simulink model "LADRC_Bloque_py"  (R2021a)
settings: Solver=ode8  StartTime=0.0  StopTime=Tsim  FixedStep=0.01  RelTol=1e-3
undefined symbols (not defined in the file or in its folder): Alpha, Kconva, Kconvp, Krad, mcecool, mcehot, mcerad, Rp, Tamb, Vfan
settings Model: Creator=djah0  LastModifiedBy=djah0
settings DataIOCC: ReturnWorkspaceOutputs=off

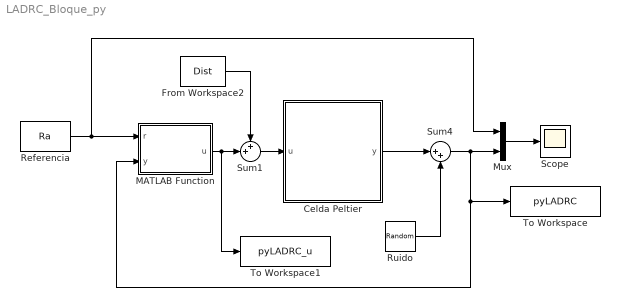
== system LADRC_Bloque_py ==
  Celda Peltier : Subsystem
  From Workspace2 : FromWorkspace  VariableName=Dist
  MATLAB Function : MATLAB Function  TreatAsAtomicUnit=on
  Mux : Mux  Inputs=2
  Referencia : FromWorkspace  VariableName=Ra
  Ruido : RandomNumber  Variance=0.002  Seed=1  SampleTime=0.2
  Scope : Scope
  Sum1 : Sum  Inputs=++|
  Sum4 : Sum  Inputs=|++
  To Workspace : ToWorkspace  VariableName=pyLADRC  SaveFormat=Timeseries  SampleTime=-1
  To Workspace1 : ToWorkspace  VariableName=pyLADRC_u  SaveFormat=Timeseries  SampleTime=-1
  wires:
  Sum1/1 -> Celda Peltier/1(u)
  MATLAB Function/1(u) -> To Workspace1/1, Sum1/2
  From Workspace2/1 -> Sum1/1
  Referencia/1 -> Mux/1, MATLAB Function/1(r)
  Mux/1 -> Scope/1
  Celda Peltier/1(y) -> Sum4/1
  Sum4/1 -> MATLAB Function/2(y), To Workspace/1, Mux/2
  Ruido/1 -> Sum4/2

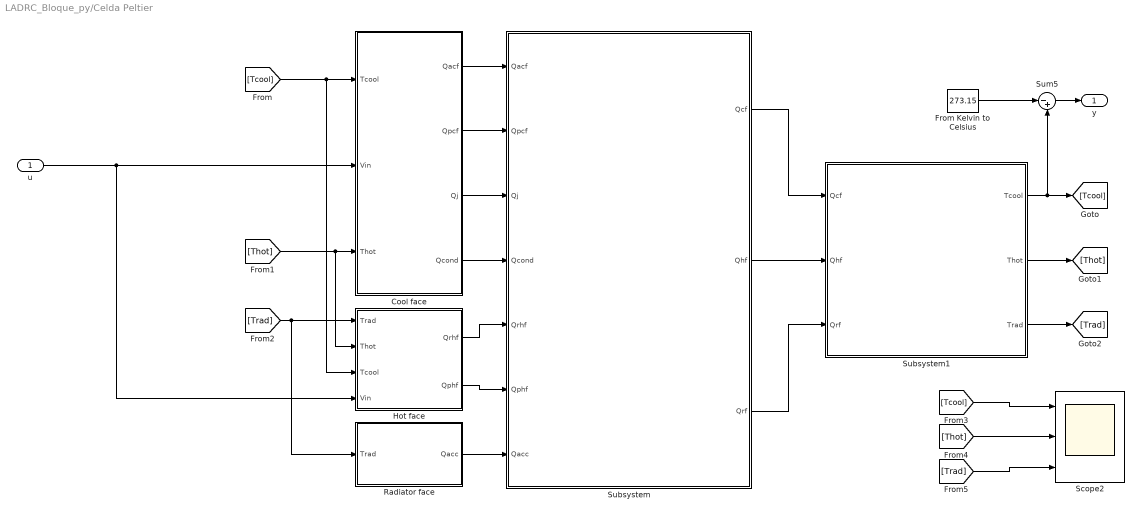
== system LADRC_Bloque_py/Celda Peltier ==
  u : Inport
  Cool face : Subsystem
  From Kelvin to Celsius : Constant  Value=273.15
  Hot face : Subsystem
  Radiator face : Subsystem
  Scope2 : Scope  NumInputPorts=3
  Subsystem : Subsystem
  Subsystem1 : Subsystem
  Sum5 : Sum  Inputs=|-+
  y : Outport  VectorParamsAs1DForOutWhenUnconnected=off
  wires:
  u/1 -> Hot face/4(Vin), Cool face/2(Vin)
  [Tcool] -> Hot face/3(Tcool), Cool face/1(Tcool)
  Subsystem1/1(Tcool) -> [Tcool], Sum5/2
  Radiator face/1(Qacc) -> Subsystem/7(Qacc)
  Subsystem1/3(Trad) -> [Trad]
  [Thot] -> Hot face/2(Thot), Cool face/3(Thot)
  [Trad] -> Hot face/1(Trad), Radiator face/1(Trad)
  Subsystem1/2(Thot) -> [Thot]
  Cool face/2(Qpcf) -> Subsystem/2(Qpcf)
  Cool face/1(Qacf) -> Subsystem/1(Qacf)
  Cool face/3(Qj) -> Subsystem/3(Qj)
  Cool face/4(Qcond) -> Subsystem/4(Qcond)
  Subsystem/1(Qcf) -> Subsystem1/1(Qcf)
  Subsystem/2(Qhf) -> Subsystem1/2(Qhf)
  Subsystem/3(Qrf) -> Subsystem1/3(Qrf)
  Hot face/1(Qrhf) -> Subsystem/5(Qrhf)
  Hot face/2(Qphf) -> Subsystem/6(Qphf)
  Sum5/1 -> y/1
  From Kelvin to Celsius/1 -> Sum5/1
  [Tcool] -> Scope2/1
  [Thot] -> Scope2/2
  [Trad] -> Scope2/3

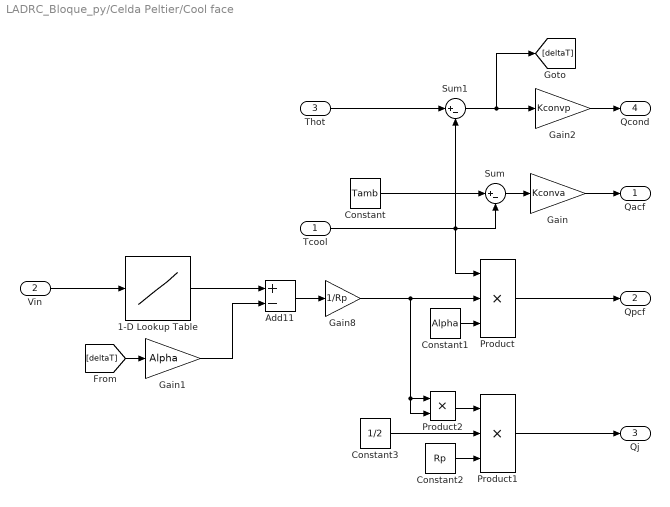
== system LADRC_Bloque_py/Celda Peltier/Cool face ==
  Tcool : Inport
  Vin : Inport  Port=2
  Thot : Inport  Port=3
  1-D Lookup Table : Lookup_n-D  NumberOfTableDimensions=1  BreakpointsForDimension1=[0,10,20,30,40,100]  Table=[0,0.625,1.378,2.138,2.891,7.23]  RndMeth=Simplest  InputSameDT=on
  Add11 : Sum  Inputs=+-
  Constant : Constant  Value=Tamb
  Constant1 : Constant  Value=Alpha
  Constant2 : Constant  Value=Rp
  Constant3 : Constant  Value=1/2
  Gain : Gain  Gain=Kconva
  Gain1 : Gain  Gain=Alpha
  Gain2 : Gain  Gain=Kconvp
  Gain8 : Gain  Gain=1/Rp
  Product : Product  Inputs=3
  Product1 : Product  Inputs=3
  Product2 : Product
  Sum : Sum  Inputs=|+-
  Sum1 : Sum  Inputs=|+-
  Qacf : Outport  VectorParamsAs1DForOutWhenUnconnected=off
  Qpcf : Outport  Port=2  VectorParamsAs1DForOutWhenUnconnected=off
  Qj : Outport  Port=3  VectorParamsAs1DForOutWhenUnconnected=off
  Qcond : Outport  Port=4  VectorParamsAs1DForOutWhenUnconnected=off
  wires:
  Constant1/1 -> Product/3
  Sum1/1 -> Gain2/1, [deltaT]
  Sum/1 -> Gain/1
  Constant/1 -> Sum/1
  Product2/1 -> Product1/1
  Constant2/1 -> Product1/3
  Constant3/1 -> Product1/2
  Tcool/1 -> Sum1/2, Product/1, Sum/2
  Gain/1 -> Qacf/1
  Gain2/1 -> Qcond/1
  Product/1 -> Qpcf/1
  Product1/1 -> Qj/1
  Thot/1 -> Sum1/1
  Vin/1 -> 1-D Lookup Table/1
  Gain8/1 -> Product2/2, Product2/1, Product/2
  Add11/1 -> Gain8/1
  1-D Lookup Table/1 -> Add11/1
  [deltaT] -> Gain1/1
  Gain1/1 -> Add11/2

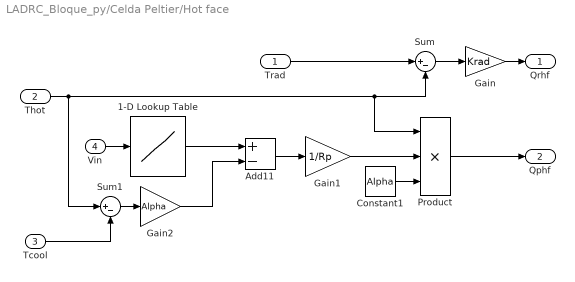
== system LADRC_Bloque_py/Celda Peltier/Hot face ==
  Trad : Inport
  Thot : Inport  Port=2
  Tcool : Inport  Port=3
  Vin : Inport  Port=4
  1-D Lookup Table : Lookup_n-D  NumberOfTableDimensions=1  BreakpointsForDimension1=[0,10,20,30,40,100]  Table=[0,0.625,1.378,2.138,2.891,7.23]  RndMeth=Simplest  InputSameDT=on
  Add11 : Sum  Inputs=+-
  Constant1 : Constant  Value=Alpha
  Gain : Gain  Gain=Krad
  Gain1 : Gain  Gain=1/Rp
  Gain2 : Gain  Gain=Alpha
  Product : Product  Inputs=3
  Sum : Sum  Inputs=|+-
  Sum1 : Sum  Inputs=|+-
  Qrhf : Outport  VectorParamsAs1DForOutWhenUnconnected=off
  Qphf : Outport  Port=2  VectorParamsAs1DForOutWhenUnconnected=off
  wires:
  Sum/1 -> Gain/1
  Trad/1 -> Sum/1
  Gain/1 -> Qrhf/1
  Thot/1 -> Sum1/1, Product/1, Sum/2
  Product/1 -> Qphf/1
  Constant1/1 -> Product/3
  Add11/1 -> Gain1/1
  1-D Lookup Table/1 -> Add11/1
  Vin/1 -> 1-D Lookup Table/1
  Gain2/1 -> Add11/2
  Gain1/1 -> Product/2
  Sum1/1 -> Gain2/1
  Tcool/1 -> Sum1/2

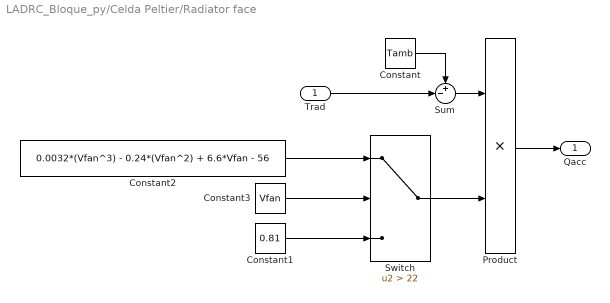
== system LADRC_Bloque_py/Celda Peltier/Radiator face ==
  Trad : Inport
  Constant : Constant  Value=Tamb
  Constant1 : Constant  Value=0.81
  Constant2 : Constant  Value=0.0032*(Vfan^3) - 0.24*(Vfan^2) + 6.6*Vfan - 56
  Constant3 : Constant  Value=Vfan
  Product : Product
  Sum : Sum  Inputs=+-|
  Switch : Switch  Criteria=u2 > Threshold  Threshold=22
  Qacc : Outport  VectorParamsAs1DForOutWhenUnconnected=off
  wires:
  Constant3/1 -> Switch/2
  Switch/1 -> Product/2
  Trad/1 -> Sum/2
  Sum/1 -> Product/1
  Product/1 -> Qacc/1
  Constant/1 -> Sum/1
  Constant2/1 -> Switch/1
  Constant1/1 -> Switch/3

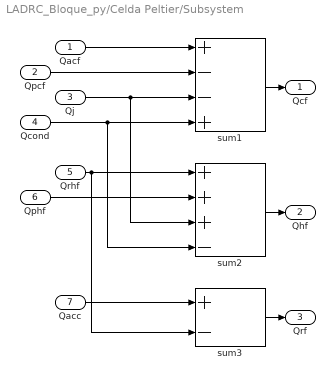
== system LADRC_Bloque_py/Celda Peltier/Subsystem ==
  Qacf : Inport
  Qpcf : Inport  Port=2
  Qj : Inport  Port=3
  Qcond : Inport  Port=4
  Qrhf : Inport  Port=5
  Qphf : Inport  Port=6
  Qacc : Inport  Port=7
  sum1 : Sum  Inputs=+--+
  sum2 : Sum  Inputs=+++-
  sum3 : Sum  Inputs=+-
  Qcf : Outport  VectorParamsAs1DForOutWhenUnconnected=off
  Qhf : Outport  Port=2  VectorParamsAs1DForOutWhenUnconnected=off
  Qrf : Outport  Port=3  VectorParamsAs1DForOutWhenUnconnected=off
  wires:
  Qcond/1 -> sum2/4, sum1/4
  Qj/1 -> sum2/3, sum1/3
  Qpcf/1 -> sum1/2
  Qacf/1 -> sum1/1
  Qrhf/1 -> sum3/2, sum2/1
  sum3/1 -> Qrf/1
  sum1/1 -> Qcf/1
  Qphf/1 -> sum2/2
  Qacc/1 -> sum3/1
  sum2/1 -> Qhf/1

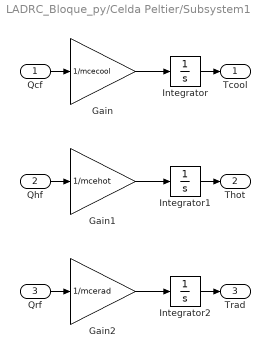
== system LADRC_Bloque_py/Celda Peltier/Subsystem1 ==
  Qcf : Inport
  Qhf : Inport  Port=2
  Qrf : Inport  Port=3
  Gain : Gain  Gain=1/mcecool
  Gain1 : Gain  Gain=1/mcehot
  Gain2 : Gain  Gain=1/mcerad
  Integrator : Integrator  InitialCondition=Tamb
  Integrator1 : Integrator  InitialCondition=Tamb
  Integrator2 : Integrator  InitialCondition=Tamb
  Tcool : Outport  VectorParamsAs1DForOutWhenUnconnected=off
  Thot : Outport  Port=2  VectorParamsAs1DForOutWhenUnconnected=off
  Trad : Outport  Port=3  VectorParamsAs1DForOutWhenUnconnected=off
  wires:
  Integrator1/1 -> Thot/1
  Gain2/1 -> Integrator2/1
  Gain1/1 -> Integrator1/1
  Qcf/1 -> Gain/1
  Integrator2/1 -> Trad/1
  Qhf/1 -> Gain1/1
  Gain/1 -> Integrator/1
  Integrator/1 -> Tcool/1
  Qrf/1 -> Gain2/1

== matlab function LADRC_Bloque_py/MATLAB Function ==
  data: r input; u output; y input
function u = pyLADRC(r, y)
%#codegen
% funciona con h = 0.03 y ode45

u = 0; % Preasignado

coder.extrinsic('pythonLADRC');

param.nx = 1;
param.b = -0.1028;
param.wc = 0.5;
param.wo = 1;
param.zo = 23.5 + 273.15;

u = pythonLADRC(r, y, param);
